simulink model "CP27E_TV"  (R2026a)
settings: Solver=ode45  StopTime=6
undefined symbols (not defined in the file or in its folder): dspblkCoreblockFVToolHelper, gcbh, P
libraries: simulink x1, slpidlib x1
settings Model: Creator=jacks  LastModifiedBy=jacks

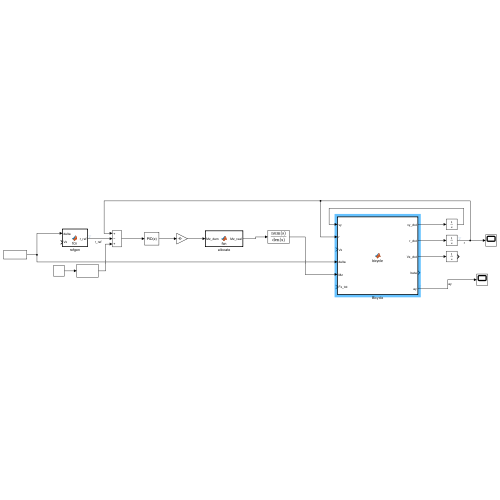
[thumbnail: Simulink's stored preview of the top-level diagram]
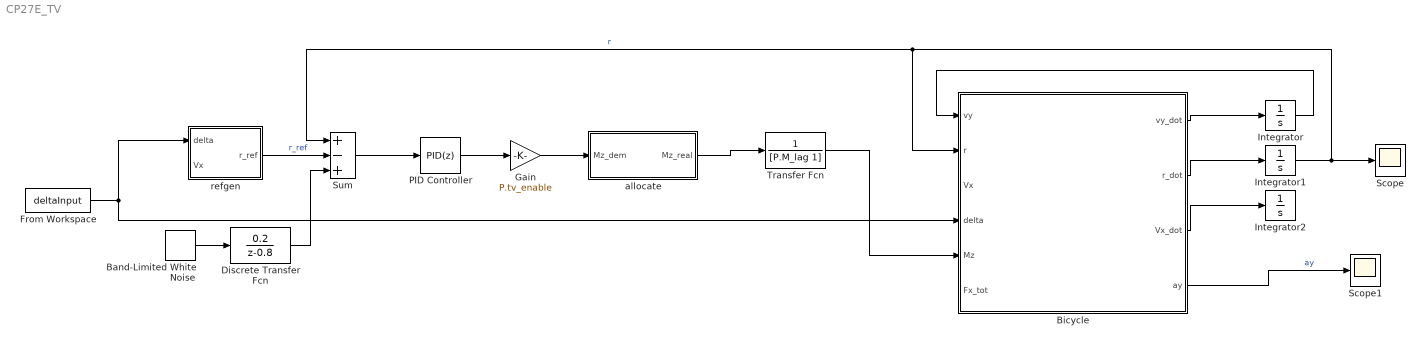
== system CP27E_TV ==
  Band-Limited White Noise : simulink/Sources/Band-Limited White Noise  Cov=1e-6  Ts=P.Ts_ctrl  seed=[23341]  VectorParams1D=off
  Bicycle : MATLAB Function  TreatAsAtomicUnit=on
  Discrete Transfer Fcn : DiscreteTransferFcn  LoadFcn=dspblkCoreblockFVToolHelper(gcbh,'load');  Numerator=[0.2]  Denominator=[1 -0.8]
      settings: CopyFcn=dspblkCoreblockFVToolHelper(gcbh,'copy');  DeleteFcn=dspblkCoreblockFVToolHelper(gcbh,'close');  ModelCloseFcn=dspblkCoreblockFVToolHelper(gcbh,'close');  PreSaveFcn=dspblkCoreblockFVToolHelper(gcbh,'presave');  PostSaveFcn=dspblkCoreblockFVToolHelper(gcbh,'postsave');  CloseFcn=dspblkCoreblockFVToolHelper(gcbh,'close');
  From Workspace : FromWorkspace  VariableName=deltaInput
  Gain : Gain  Gain=P.tv_enable
  Integrator : Integrator
  Integrator1 : Integrator
  Integrator2 : Integrator
  PID Controller : slpidlib/PID Controller  Controller=PID  Form=Parallel  TimeDomain=Discrete-time  UseExternalTs=off  SampleTime=P.Ts_ctrl  IntegratorMethod=Forward Euler  FilterMethod=Forward Euler  ControllerParametersSource=internal  P=P.Kp  I=P.Ki  UseKiTs=off  D=P.Kd  UseExternalDerivativeSource=off  N=100  UseFilter=off  TunerSelectOption=Transfer Function Based (PID Tuner App)  InitialConditionSource=internal  InitialConditionForIntegrator=0  InitialConditionForFilter=0  DifferentiatorICPrevScaledInput=0  ExternalReset=none  TrackingMode=off  Kt=1  LimitOutput=off  SatLimitsSource=internal  UpperSaturationLimit=inf  LowerSaturationLimit=-inf  LinearizeAsGain=on  AntiWindupMode=none  Kb=1  LimitIntegrator=off  UpperIntegratorSaturationLimit=inf  LowerIntegratorSaturationLimit=-inf  POutMin=[]  POutMax=[]  IOutMin=[]  IOutMax=[]  DOutMin=[]  DOutMax=[]  NOutMin=[]  NOutMax=[]  SumOutMin=[]  SumOutMax=[]  SaturationOutMin=[]  SaturationOutMax=[]  PParamMin=[]  PParamMax=[]  IParamMin=[]  IParamMax=[]  DParamMin=[]  DParamMax=[]  NParamMin=[]  NParamMax=[]  KbParamMin=[]  KbParamMax=[]  KtParamMin=[]  KtParamMax=[]  KbOutMin=[]  KbOutMax=[]  KtOutMin=[]  KtOutMax=[]  IntegratorOutMin=[]  IntegratorOutMax=[]  FilterOutMin=[]  FilterOutMax=[]  SumI1OutMin=[]  SumI1OutMax=[]  SumI2OutMin=[]  SumI2OutMax=[]  SumI3OutMin=[]  SumI3OutMax=[]  SumI4OutMin=[]  SumI4OutMax=[]  SumDOutMin=[]  SumDOutMax=[]  DifferentiatorOutMin=[]  DifferentiatorOutMax=[]  FilterDiffOutCoefMin=[]  FilterDiffOutCoefMax=[]  ReciprocalOutMin=[]  ReciprocalOutMax=[]  SumDenOutMin=[]  SumDenOutMax=[]  SumNumOutMin=[]  SumNumOutMax=[]  DivideOutMin=[]  DivideOutMax=[]  UdiffTsProdOutMin=[]  UdiffTsProdOutMax=[]  NTsProdOutMin=[]  NTsProdOutMax=[]  UintegralTsProdOutMin=[]  UintegralTsProdOutMax=[]  UngainTsProdOutMin=[]  UngainTsProdOutMax=[]  ClampingZeroOutDataTypeStr=Inherit: Inherit via back propagation  ClampingZeroOutMin=[]  ClampingZeroOutMax=[]  FilterDenConstantOutDataTypeStr=Inherit: Inherit via back propagation  FilterDenConstantOutMin=[]  FilterDenConstantOutMax=[]  PCopyOutDataTypeStr=Inherit: Inherit via back propagation  PCopyOutMin=[]  PCopyOutMax=[]  NCopyOutDataTypeStr=Inherit: Inherit via back propagation  NCopyOutMin=[]  NCopyOutMax=[]  IntegratorContinuousStateAttributes=''  IntegratorStateMustResolveToSignalObject=off  IntegratorRTWStateStorageClass=Auto  FilterContinuousStateAttributes=''  FilterStateMustResolveToSignalObject=off  FilterRTWStateStorageClass=Auto  ParallelPVariant=InternalParameters  IdealPVariant=Disabled  IVariant=InternalParameters  DVariant=InternalParameters  IntegratorVariant=Discrete  SatVariant=Disabled  AWVariant=Passthrough  PCopyVariant=Disabled  TRVariant=Disabled  FdbkBlocksVariant=Forward  IdealPFdbkVariant=Disabled  SatFdbkVariant=Disabled  DerivativeFilterVariant=Differentiator  NVariant=Passthrough  NCopyVariant=Disabled_SignalSpec  FilterICVariant=InternalICsDifferentiator  IntegratorICVariant=InternalICs  ExternalResetVariant=Disabled  TRSumVariant=Passthrough  SumFdbkVariant=Disabled  SumVariant=Sum_PID  TsampFilterVariant=InternalTs  TsampNgainVariant=Passthrough  TsampIntegralVariant=Disabled_SignalSpec  ExternalSaturationOutDataTypeStr=Inherit: Same as second input  DerivativeSourceVariant=ErrorSignal  PreIntVariant=InternalPreInt
  Scope : Scope
      settings: ActiveDisplayYMinimum=-0.83562446557997683  ActiveDisplayYMaximum=0.89552647021979792
  Scope1 : Scope
  Sum : Sum  Inputs=+-+
  Transfer Fcn : TransferFcn  Denominator=[P.M_lag 1]
  allocate : MATLAB Function  TreatAsAtomicUnit=on
  refgen : MATLAB Function  TreatAsAtomicUnit=on
  wires:
  Bicycle/1(vy_dot) -> Integrator/1
  Integrator/1 -> Bicycle/1(vy)
  Bicycle/2(r_dot) -> Integrator1/1
  Integrator1/1 -> Scope/1, Bicycle/2(r), Sum/1  "r"
  From Workspace/1 -> refgen/1(delta), Bicycle/4(delta)
  refgen/1(r_ref) -> Sum/2  "r_ref"
  Sum/1 -> PID Controller/1
  PID Controller/1 -> Gain/1
  Gain/1 -> allocate/1(Mz_dem)
  allocate/1(Mz_real) -> Transfer Fcn/1
  Bicycle/4(ay) -> Scope1/1  "ay"
  Transfer Fcn/1 -> Bicycle/5(Mz)
  Band-Limited White Noise/1 -> Discrete Transfer Fcn/1
  Discrete Transfer Fcn/1 -> Sum/3
  Bicycle/3(Vx_dot) -> Integrator2/1

== matlab function CP27E_TV/refgen ==
  data: delta input; r_ref output; Vx input; P parameter
function r_ref = fcn(delta, Vx, P)
    r_ref = refgen(delta, Vx, P);
end

== matlab function CP27E_TV/Bicycle ==
  data: vy input; vy_dot output; r input; Vx input; delta input; Mz input; Fx_tot input; r_dot output; Vx_dot output; ay output; P parameter
function [vy_dot, r_dot, Vx_dot, ay] = bicycle(vy, r, Vx, delta, Mz, Fx_tot, P)
    [vy_dot, r_dot, Vx_dot, beta, ay] = bicycle(vy, r, Vx, delta, Mz, Fx_tot, P);
end

== matlab function CP27E_TV/allocate ==
  data: Mz_dem input; Mz_real output; P parameter
function Mz_real = fcn(Mz_dem, P)
    [~,~,~,~,Mz_real,~] = allocate(Mz_dem, P.T_drive, P);
end
